simulink model "cuantizador2"  (R2015a)
settings: Solver=ode45  StartTime=0.0  StopTime=2.0  RelTol=1e-3
settings Model: Creator=hppoc  LastModifiedBy=hppoc

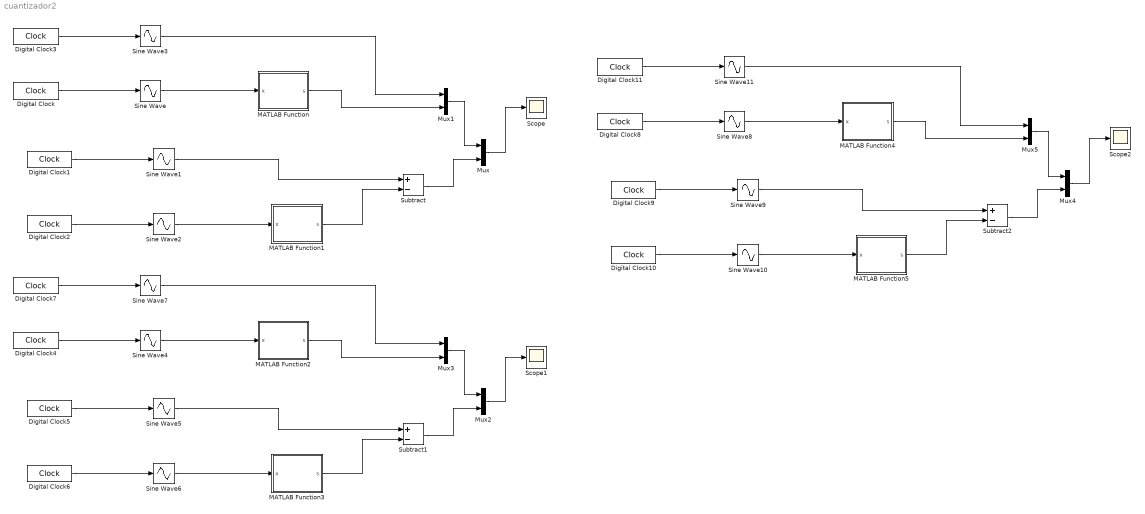
== system cuantizador2 ==
  Digital Clock{,1..11} (12 alike) : DigitalClock  SampleTime=0.001
  MATLAB Function : MATLAB Function  RequirementInfo="{}  %GIDa_527a6e52_c067_4402_b98e_86dba84f34dc"  TreatAsAtomicUnit=on
  MATLAB Function1 : MATLAB Function  RequirementInfo={} %GIDa_fd8e49f6_3079_412f_81b4_a0016d358ead  TreatAsAtomicUnit=on
  MATLAB Function2 : MATLAB Function  RequirementInfo={} %GIDa_d5a3f87e_0c75_4765_8eec_b5d2f3b8c74e  TreatAsAtomicUnit=on
  MATLAB Function3 : MATLAB Function  RequirementInfo={} %GIDa_3233024f_fded_4842_aa0b_fe82489d8ddf  TreatAsAtomicUnit=on
  MATLAB Function4 : MATLAB Function  RequirementInfo={} %GIDa_80c91e5f_28f4_4b5d_bf2b_2f72b3352565  TreatAsAtomicUnit=on
  MATLAB Function5 : MATLAB Function  RequirementInfo={} %GIDa_fc5a48f9_1031_4f7d_96d9_feea33fd816a  TreatAsAtomicUnit=on
  Mux{,1..5} (6 alike) : Mux  Inputs=2
  Scope : Scope
      settings: YMin=-1  YMax=1
  Scope1 : Scope
      settings: YMin=-1  YMax=1
  Scope2 : Scope
      settings: YMin=-1  YMax=1  SaveName=ScopeData2
  Sine Wave{,1..11} (12 alike) : Sin  SineType=Sample based  TimeSource=Use external signal  Frequency=2*pi  Samples=1000  SampleTime=0
  Subtract : Sum  Inputs=+-
  Subtract1 : Sum  Inputs=+-
  Subtract2 : Sum  Inputs=+-
  wires:
  Digital Clock/1 -> Sine Wave/1
  Mux/1 -> Scope/1
  Sine Wave/1 -> MATLAB Function/1(x)
  Subtract/1 -> Mux/2
  Digital Clock1/1 -> Sine Wave1/1
  Sine Wave1/1 -> Subtract/1
  Digital Clock2/1 -> Sine Wave2/1
  Sine Wave2/1 -> MATLAB Function1/1(x)
  MATLAB Function1/1(s) -> Subtract/2
  Digital Clock3/1 -> Sine Wave3/1
  Sine Wave3/1 -> Mux1/1
  MATLAB Function/1(s) -> Mux1/2
  Mux1/1 -> Mux/1
  Digital Clock4/1 -> Sine Wave4/1
  Mux2/1 -> Scope1/1
  Sine Wave4/1 -> MATLAB Function2/1(x)
  Subtract1/1 -> Mux2/2
  Digital Clock5/1 -> Sine Wave5/1
  Sine Wave5/1 -> Subtract1/1
  Digital Clock6/1 -> Sine Wave6/1
  Sine Wave6/1 -> MATLAB Function3/1(x)
  MATLAB Function3/1(s) -> Subtract1/2
  Digital Clock7/1 -> Sine Wave7/1
  Sine Wave7/1 -> Mux3/1
  MATLAB Function2/1(s) -> Mux3/2
  Mux3/1 -> Mux2/1
  Digital Clock8/1 -> Sine Wave8/1
  Mux4/1 -> Scope2/1
  Sine Wave8/1 -> MATLAB Function4/1(x)
  Subtract2/1 -> Mux4/2
  Digital Clock9/1 -> Sine Wave9/1
  Sine Wave9/1 -> Subtract2/1
  Digital Clock10/1 -> Sine Wave10/1
  Sine Wave10/1 -> MATLAB Function5/1(x)
  MATLAB Function5/1(s) -> Subtract2/2
  Digital Clock11/1 -> Sine Wave11/1
  Sine Wave11/1 -> Mux5/1
  MATLAB Function4/1(s) -> Mux5/2
  Mux5/1 -> Mux4/1

== matlab function cuantizador2/MATLAB Function1 ==
  data: s output; x input
function s=cuantizador(x)
    l=8;
    Xmax=1;
    Escalon=(2*Xmax)/l;
    y=zeros(1,l+1);
    y(1)=-Xmax;
    for i=1:l
        y(i+1)=y(i)+Escalon;
    end
    Y=zeros(1,l);
    for i=1:l
        Y(i)=(y(i)+y(i+1))/2;
    end
    aux=y(1);
    senal=0;
    for i=1:length(y)
        if(x>=y(length(y)))
            senal=Y(length(Y));
        elseif(x<=y(1))
            senal=Y(1);
        elseif(x>=y(i)&&x<y(i+1))
            senal=Y(i);
        end
    end
    s=senal;

== matlab function cuantizador2/MATLAB Function ==
  data: s output; x input
function s=cuantizador(x)
    l=8;
    Xmax=1;
    Escalon=(2*Xmax)/l;
    y=zeros(1,l+1);
    y(1)=-Xmax;
    for i=1:l
        y(i+1)=y(i)+Escalon;
    end
    Y=zeros(1,l);
    for i=1:l
        Y(i)=(y(i)+y(i+1))/2;
    end
    aux=y(1);
    senal=0;
    for i=1:length(y)
        if(x>=y(length(y)))
            senal=Y(length(Y));
        elseif(x<=y(1))
            senal=Y(1);
        elseif(x>=y(i)&&x<y(i+1))
            senal=Y(i);
        end
    end
    s=senal;

== matlab function cuantizador2/MATLAB Function2 ==
  data: s output; x input
function s=cuantizador(x)
    l=16;
    Xmax=1;
    Escalon=(2*Xmax)/l;
    y=zeros(1,l+1);
    y(1)=-Xmax;
    for i=1:l
        y(i+1)=y(i)+Escalon;
    end
    Y=zeros(1,l);
    for i=1:l
        Y(i)=(y(i)+y(i+1))/2;
    end
    aux=y(1);
    senal=0;
    for i=1:length(y)
        if(x>=y(length(y)))
            senal=Y(length(Y));
        elseif(x<=y(1))
            senal=Y(1);
        elseif(x>=y(i)&&x<y(i+1))
            senal=Y(i);
        end
    end
    s=senal;

== matlab function cuantizador2/MATLAB Function3 ==
  data: s output; x input
function s=cuantizador(x)
    l=16;
    Xmax=1;
    Escalon=(2*Xmax)/l;
    y=zeros(1,l+1);
    y(1)=-Xmax;
    for i=1:l
        y(i+1)=y(i)+Escalon;
    end
    Y=zeros(1,l);
    for i=1:l
        Y(i)=(y(i)+y(i+1))/2;
    end
    aux=y(1);
    senal=0;
    for i=1:length(y)
        if(x>=y(length(y)))
            senal=Y(length(Y));
        elseif(x<=y(1))
            senal=Y(1);
        elseif(x>=y(i)&&x<y(i+1))
            senal=Y(i);
        end
    end
    s=senal;

== matlab function cuantizador2/MATLAB Function4 ==
  data: s output; x input
function s=cuantizador(x)
    l=32;
    Xmax=1;
    Escalon=(2*Xmax)/l;
    y=zeros(1,l+1);
    y(1)=-Xmax;
    for i=1:l
        y(i+1)=y(i)+Escalon;
    end
    Y=zeros(1,l);
    for i=1:l
        Y(i)=(y(i)+y(i+1))/2;
    end
    aux=y(1);
    senal=0;
    for i=1:length(y)
        if(x>=y(length(y)))
            senal=Y(length(Y));
        elseif(x<=y(1))
            senal=Y(1);
        elseif(x>=y(i)&&x<y(i+1))
            senal=Y(i);
        end
    end
    s=senal;

== matlab function cuantizador2/MATLAB Function5 ==
  data: s output; x input
function s=cuantizador(x)
    l=32;
    Xmax=1;
    Escalon=(2*Xmax)/l;
    y=zeros(1,l+1);
    y(1)=-Xmax;
    for i=1:l
        y(i+1)=y(i)+Escalon;
    end
    Y=zeros(1,l);
    for i=1:l
        Y(i)=(y(i)+y(i+1))/2;
    end
    aux=y(1);
    senal=0;
    for i=1:length(y)
        if(x>=y(length(y)))
            senal=Y(length(Y));
        elseif(x<=y(1))
            senal=Y(1);
        elseif(x>=y(i)&&x<y(i+1))
            senal=Y(i);
        end
    end
    s=senal;
